simulink model "D_20210914_Modell_Inbetriebnahme_BreakOutBox_Jetson"  (R2021a)
settings: Solver=ode1  StartTime=0.0  StopTime=500  FixedStep=Ts  RelTol=1e-3
PreLoadFcn:
  | pulsePeriod = 0.05;
  | 
  | Ts = 0.001;
  | 
  | FPGA_Frequency = 75000000;
  | 
  | ts_IO691 = 5e-3;
PostLoadFcn:
  | ewolfSetUp
InitFcn:
  | pulsePeriod = 0.05;
  | 
  | Ts = 0.001;
  | 
  | FPGA_Frequency = 75000000;
  | 
  | ts_IO691 = 5e-3;
StopFcn:
  | Simulink.sdi.clearPreferences;
  | if isfile(['sdi_view_',bdroot,'.mldatx'])
  | Simulink.sdi.view;
  | pause(3);
  | Simulink.sdi.loadView(['sdi_view_',bdroot,]);
  | end
values from neighbouring files (symbols this model uses):
  max_ac = 2    [ewolfSetUp.m]
  max_steer = 0.26    [ewolfSetUp.m]
  min_ac = -3    [ewolfSetUp.m]
  min_steer = -0.26    [ewolfSetUp.m]
  PredictionHorizon = 30    [ewolfSetUp.m]
undefined symbols (not defined in the file or in its folder): canChannel, DiscIntNeverNeededParam, Ended, HS, IO291, IO397, Single
libraries: lllalib x255, canmsglib x143, simulink x33, speedgoatlib_IO191 x5, speedgoatlib_IO291 x5, speedgoatlib_IO691 x3, slrealtimeiplib x2, simulink_extras x1, speedgoatlib_fpga_dio x1, speedgoatlib_fpga_quadrature x1, speedgoatlib_fpga x1, canlib x1
(part 2 of 7)

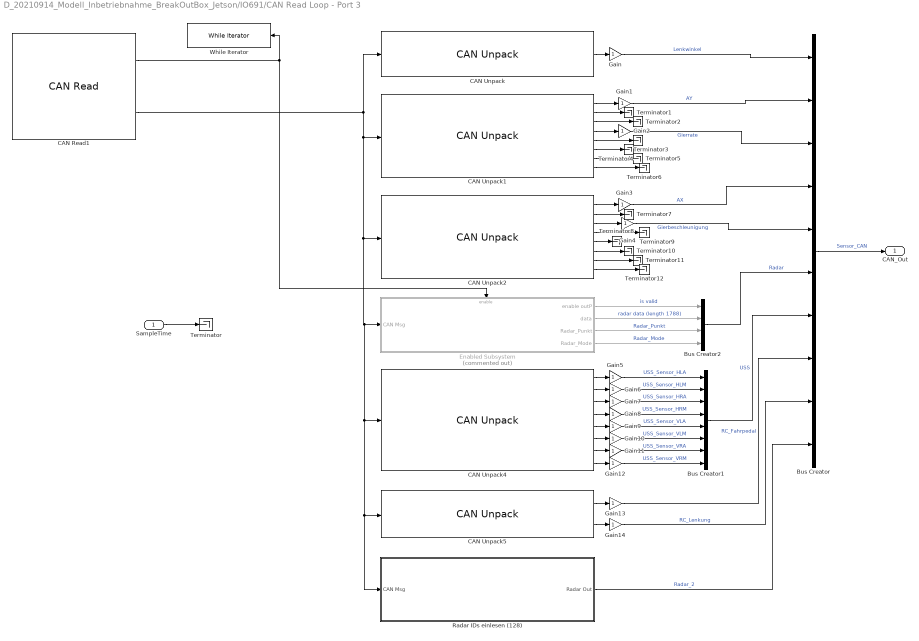
== system D_20210914_Modell_Inbetriebnahme_BreakOutBox_Jetson/IO691/CAN Read Loop - Port 3 ==
  SampleTime : Inport
  Bus Creator : BusCreator  Inputs=10
  Bus Creator1 : BusCreator  Inputs=8
  Bus Creator2 : BusCreator  Inputs=4
  CAN Read1 : speedgoatlib_IO691/CAN Read  id=1  ts=-1  channel=1  messageType=CAN  canType=CAN (HS)  BusOutput=off  initValues=[691 1 -1 0 1 1 0]
      settings: SourceProductName=Simulink Real-Time: Speedgoat Library
  CAN Unpack : canmsglib/CAN Unpack  CANdbFile=eWolf_SensorCAN.dbc  MsgList=Lenkwinkelsensor  MsgName=Lenkwinkelsensor  MsgIDType=Standard (11-bit identifier)  MsgIdentifier=2  MsgLength=2  SignalInfo={'Lenkwinkel','0','16','LE','signed','Standard','0','0.09882','0','-630','630'}  IDPort=off  TimestampPort=off  ErrorPort=off  RemotePort=off  LengthPort=off  StatusPort=off  ApplyMinMax=off
      settings: SourceProductBaseCode=ME,XP,VN  DataFormat=CANdb specified signals
  CAN Unpack1 : canmsglib/CAN Unpack  CANdbFile=eWolf_SensorCAN.dbc  MsgList=Beschleunigungssensor  MsgName=Beschleunigungssensor  MsgIDType=Standard (11-bit identifier)  MsgIdentifier=304  MsgLength=8  SignalInfo={'AY1','32','16','LE','unsigned','Standard','0','0.0001274','-4.1768','-4.1768','4.1768';'AY1_STAT','48','4','LE','unsigned','Standard','0','1','0','0','15';'CLU_STAT','16','4','LE','unsigned','Standard','0','1','0','0','15';'Gierrate','0','16','LE','unsigned','Standard','0','0.005','-163.84','-163.84','163.84';'Gierrate_STAT','52','4','LE','unsigned','Standard','0','1','0','0','15';'PSIP1_EXT_STAT','24','8','LE','unsigned','Standard','0','1','0','0','255';'TX1_CRC','56','8','LE','unsigned','Standard','0','1','0','0','255';'TX1_MSG_CNT','20','4','LE','unsigned','Standard','0','1','0','0','15'}  IDPort=off  TimestampPort=off  ErrorPort=off  RemotePort=off  LengthPort=off  StatusPort=off  ApplyMinMax=off
      settings: SourceProductBaseCode=ME,XP,VN  DataFormat=CANdb specified signals
  CAN Unpack2 : canmsglib/CAN Unpack  CANdbFile=eWolf_SensorCAN.dbc  MsgList=Beschleunigungssensor_2  MsgName=Beschleunigungssensor_2  MsgIDType=Standard (11-bit identifier)  MsgIdentifier=305  MsgLength=8  SignalInfo={'AX1','32','16','LE','unsigned','Standard','0','0.0001274','-4.1768','-4.1768','4.1768';'AX1_STAT','52','4','LE','unsigned','Standard','0','1','0','0','15';'Gierbeschleunigung','0','16','LE','unsigned','Standard','0','0.125','-4096','-4096','4096';'Gierbeschleunigung_STAT','20','4','LE','unsigned','Standard','0','1','0','0','15';'TX2_CRC','56','8','LE','unsigned','Standard','0','1','0','0','255';'TX2_MSG_CNT','48','4','LE','unsigned','Standard','0','1','0','0','15';'TX2_RES1','16','4','LE','unsigned','Standard','0','1','0','0','15';'TX2_RES2','24','8','LE','unsigned','Standard','0','1','0','0','255'}  IDPort=off  TimestampPort=off  ErrorPort=off  RemotePort=off  LengthPort=off  StatusPort=off  ApplyMinMax=off
      settings: SourceProductBaseCode=ME,XP,VN  DataFormat=CANdb specified signals
  CAN Unpack4 : canmsglib/CAN Unpack  CANdbFile=eWolf_SensorCAN.dbc  MsgList=Ultraschallsystem  MsgName=Ultraschallsystem  MsgIDType=Standard (11-bit identifier)  MsgIdentifier=16  MsgLength=8  SignalInfo={'USS_Sensor_HLA','32','8','LE','unsigned','Standard','0','1','0','0','255';'USS_Sensor_HLM','40','8','LE','unsigned','Standard','0','1','0','0','255';'USS_Sensor_HRA','56','8','LE','unsigned','Standard','0','1','0','0','255';'USS_Sensor_HRM','48','8','LE','unsigned','Standard','0','1','0','0','255';'USS_Sensor_VLA','0','8','LE','unsigned','Standard','0','1','0','0','255';'USS_Sensor_VLM','8','8','LE','unsigned','Standard','0','1','0','0','255';'USS_Sensor_VRA','24','8','LE','unsigned','Standard','0','1','0','0','255';'USS_Sensor_VRM','16','8','LE','unsigned','Standard','0','1','0','0','255'}  IDPort=off  TimestampPort=off  ErrorPort=off  RemotePort=off  LengthPort=off  StatusPort=off  ApplyMinMax=off
      settings: SourceProductBaseCode=ME,XP,VN  DataFormat=CANdb specified signals
  CAN Unpack5 : canmsglib/CAN Unpack  CANdbFile=eWolf_SensorCAN.dbc  MsgList=RC_Fernsteuerung  MsgName=RC_Fernsteuerung  MsgIDType=Standard (11-bit identifier)  MsgIdentifier=17  MsgLength=2  SignalInfo={'RC_Fahrpedal','8','8','LE','unsigned','Standard','0','1','0','0','255';'RC_Lenkung','0','8','LE','unsigned','Standard','0','1','0','0','255'}  IDPort=off  TimestampPort=off  ErrorPort=off  RemotePort=off  LengthPort=off  StatusPort=off  ApplyMinMax=off
      settings: SourceProductBaseCode=ME,XP,VN  DataFormat=CANdb specified signals
  Enabled Subsystem : Subsystem  Commented=on  TreatAsAtomicUnit=on
  Gain{,1..14} (15 alike) : Gain
  Radar IDs einlesen (128) : Subsystem
  Terminator{,1..12} (13 alike) : Terminator
  While Iterator : WhileIterator  MaxIters=501  WhileBlockType=do-while
  CAN_Out : Outport
  wires:
  SampleTime/1 -> Terminator/1
  CAN Read1/1 -> Enabled Subsystem/Enable, While Iterator/1
  CAN Read1/2 -> CAN Unpack/1, Radar IDs einlesen (128)/1(CAN Msg), CAN Unpack5/1, CAN Unpack4/1, Enabled Subsystem/1(CAN Msg), CAN Unpack2/1, CAN Unpack1/1
  Bus Creator/1 -> CAN_Out/1  "Sensor_CAN"
  CAN Unpack/1 -> Gain/1
  CAN Unpack1/1 -> Gain1/1
  CAN Unpack1/5 -> Terminator3/1
  CAN Unpack2/1 -> Gain3/1
  CAN Unpack2/5 -> Terminator8/1
  CAN Unpack1/2 -> Terminator1/1
  CAN Unpack1/3 -> Terminator2/1
  CAN Unpack1/4 -> Gain2/1
  CAN Unpack1/6 -> Terminator4/1
  CAN Unpack1/7 -> Terminator5/1
  CAN Unpack1/8 -> Terminator6/1
  Gain/1 -> Bus Creator/1  "Lenkwinkel"
  Gain1/1 -> Bus Creator/2  "AY"
  Gain2/1 -> Bus Creator/3  "Gierrate"
  Gain3/1 -> Bus Creator/4  "AX"
  Gain4/1 -> Bus Creator/5  "Gierbeschleunigung"
  CAN Unpack2/2 -> Terminator7/1
  CAN Unpack2/3 -> Gain4/1
  CAN Unpack2/4 -> Terminator9/1
  CAN Unpack2/6 -> Terminator10/1
  CAN Unpack2/7 -> Terminator11/1
  CAN Unpack2/8 -> Terminator12/1
  CAN Unpack4/1 -> Gain5/1
  CAN Unpack4/2 -> Gain6/1
  CAN Unpack4/3 -> Gain7/1
  CAN Unpack4/4 -> Gain8/1
  CAN Unpack4/5 -> Gain9/1
  CAN Unpack4/6 -> Gain10/1
  CAN Unpack4/7 -> Gain11/1
  CAN Unpack4/8 -> Gain12/1
  Gain5/1 -> Bus Creator1/1  "USS_Sensor_HLA"
  Gain6/1 -> Bus Creator1/2  "USS_Sensor_HLM"
  Gain7/1 -> Bus Creator1/3  "USS_Sensor_HRA"
  Gain8/1 -> Bus Creator1/4  "USS_Sensor_HRM"
  Gain9/1 -> Bus Creator1/5  "USS_Sensor_VLA"
  Gain10/1 -> Bus Creator1/6  "USS_Sensor_VLM"
  Gain11/1 -> Bus Creator1/7  "USS_Sensor_VRA"
  Gain12/1 -> Bus Creator1/8  "USS_Sensor_VRM"
  Bus Creator1/1 -> Bus Creator/7  "USS"
  CAN Unpack5/1 -> Gain13/1
  CAN Unpack5/2 -> Gain14/1
  Gain13/1 -> Bus Creator/8  "RC_Fahrpedal"
  Gain14/1 -> Bus Creator/9  "RC_Lenkung"
  Enabled Subsystem/1(enable outP) -> Bus Creator2/1  "is valid"
  Enabled Subsystem/2(data) -> Bus Creator2/2  "radar data (length 1788)"
  Enabled Subsystem/3(Radar_Punkt) -> Bus Creator2/3  "Radar_Punkt"
  Enabled Subsystem/4(Radar_Mode) -> Bus Creator2/4  "Radar_Mode"
  Bus Creator2/1 -> Bus Creator/6  "Radar"
  Radar IDs einlesen (128)/1(Radar Out) -> Bus Creator/10  "Radar_2"

== system D_20210914_Modell_Inbetriebnahme_BreakOutBox_Jetson/Nvidia_Jetson/LaneFollowingAndControl ==
  Set velocity : Inport
  Longitudinal_Velocity : Inport  Port=2
  Lane Detections : Inport  Port=3
  Estimate Lane Center1 : Subsystem  VariantControl=v2
  MPC Controller : Subsystem
  steering_angle : Outport
  acceleration : Outport  Port=2
  wires:
  Longitudinal_Velocity/1 -> MPC Controller/2(Longitudinal velocity), Estimate Lane Center1/2(Longitudinal Velocity)
  MPC Controller/2(Acceleration) -> acceleration/1  "acceleration"
  Estimate Lane Center1/2(Lateral Offset) -> MPC Controller/4(Lateral deviation)  "lateral_deviation"
  Estimate Lane Center1/1(Previewed Curvature) -> MPC Controller/3(Curvature)  "previewed_curvature"
  Estimate Lane Center1/3(Heading Angle) -> MPC Controller/5(Relative yaw angle)  "relative_yaw_angle"
  Set velocity/1 -> MPC Controller/1(Set velocity)
  MPC Controller/1(Steering Angle) -> steering_angle/1  "steering_angle"
  Lane Detections/1 -> Estimate Lane Center1/1(Lane Detections)

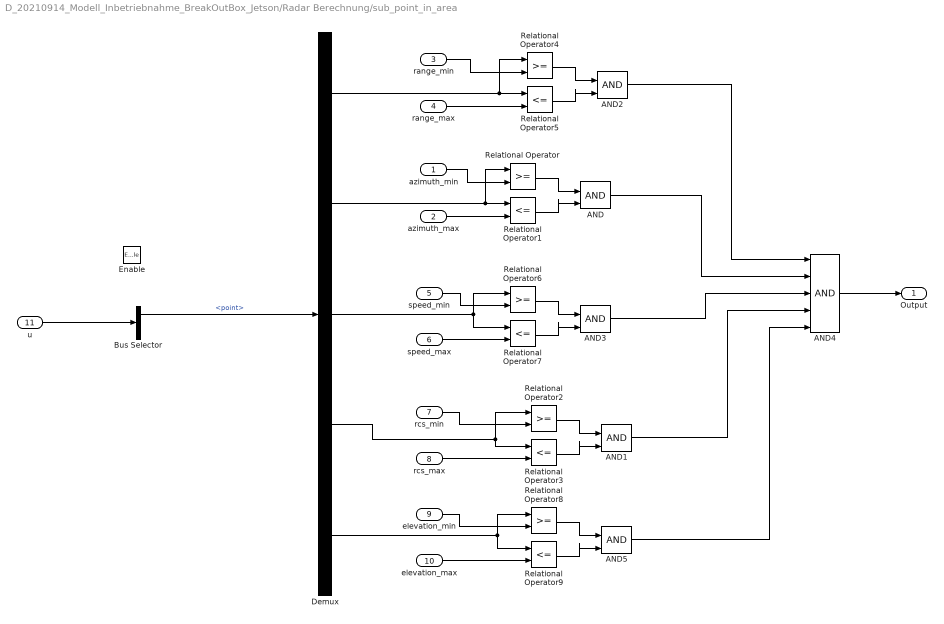
== system D_20210914_Modell_Inbetriebnahme_BreakOutBox_Jetson/Radar Berechnung/sub_point_in_area ==
  azimuth_min : Inport
  azimuth_max : Inport  Port=2
  range_min : Inport  Port=3
  range_max : Inport  Port=4
  speed_min : Inport  Port=5
  speed_max : Inport  Port=6
  rcs_min : Inport  Port=7
  rcs_max : Inport  Port=8
  elevation_min : Inport  Port=9
  elevation_max : Inport  Port=10
  u : Inport  Port=11
  Enable : EnablePort
  AND{,1..3,5} (5 alike) : Logic  IconShape=distinctive  AllPortsSameDT=off  OutDataTypeStr=boolean
  AND4 : Logic  Inputs=5  IconShape=distinctive  AllPortsSameDT=off  OutDataTypeStr=boolean
  Bus Selector : BusSelector  OutputSignals=point,CANID
  Demux : Demux  Outputs=5
  Relational Operator{,2,4,6,8} (5 alike) : RelationalOperator  OutDataTypeStr=boolean  RndMeth=Simplest
  Relational Operator{1,3,5,7,9} (5 alike) : RelationalOperator  Operator=<=  OutDataTypeStr=boolean  RndMeth=Simplest
  Output : Outport
  wires:
  Demux/5 -> Relational Operator8/1, Relational Operator9/1
  Demux/4 -> Relational Operator3/1, Relational Operator2/1
  Demux/3 -> Relational Operator6/1, Relational Operator7/1
  Demux/1 -> Relational Operator5/1, Relational Operator4/1
  Demux/2 -> Relational Operator1/1, Relational Operator/1
  elevation_max/1 -> Relational Operator9/2
  AND5/1 -> AND4/5
  Relational Operator8/1 -> AND5/1
  Relational Operator9/1 -> AND5/2
  elevation_min/1 -> Relational Operator8/2
  range_min/1 -> Relational Operator4/2
  azimuth_min/1 -> Relational Operator/2
  speed_min/1 -> Relational Operator6/2
  rcs_min/1 -> Relational Operator2/2
  Relational Operator6/1 -> AND3/1
  Relational Operator/1 -> AND/1
  AND4/1 -> Output/1
  Relational Operator4/1 -> AND2/1
  Relational Operator2/1 -> AND1/1
  Relational Operator5/1 -> AND2/2
  Relational Operator3/1 -> AND1/2
  Relational Operator7/1 -> AND3/2
  speed_max/1 -> Relational Operator7/2
  Relational Operator1/1 -> AND/2
  AND2/1 -> AND4/1
  u/1 -> Bus Selector/1
  AND/1 -> AND4/2
  AND1/1 -> AND4/4
  Bus Selector/1 -> Demux/1  "<point>"
  rcs_max/1 -> Relational Operator3/2
  range_max/1 -> Relational Operator5/2
  AND3/1 -> AND4/3
  azimuth_max/1 -> Relational Operator1/2

== system D_20210914_Modell_Inbetriebnahme_BreakOutBox_Jetson/Bremspedal Steuerung/QAD Steuerung1/Anti-Relaisprellen ==
  In : Inport
  Bias : Bias  Bias=-Ts
  Compare To Zero : simulink/Logic and Bit Operations/Compare To Zero  relop===  OutDataTypeStr=boolean
  Constant : Constant  Value=0.2
  Constant1 : Constant  Value=0
  Delay1 : Delay  DelayLength=1  InputProcessing=Columns as channels (frame based)
  Detect Increase : simulink/Logic and Bit Operations/Detect Increase  vinit=0.0  OutDataTypeStr=boolean
  Saturation : Saturate  UpperLimit=0.2  LowerLimit=0
  Switch : Switch  Criteria=u2 ~= 0
  Switch1 : Switch  Criteria=u2 ~= 0
  Out : Outport  VectorParamsAs1DForOutWhenUnconnected=off
  wires:
  Compare To Zero/1 -> Switch1/2
  In/1 -> Detect Increase/1, Switch1/1
  Switch1/1 -> Out/1
  Constant1/1 -> Switch1/3
  Delay1/1 -> Bias/1, Compare To Zero/1
  Constant/1 -> Switch/1
  Detect Increase/1 -> Switch/2
  Switch/1 -> Delay1/1
  Bias/1 -> Saturation/1
  Saturation/1 -> Switch/3

== system D_20210914_Modell_Inbetriebnahme_BreakOutBox_Jetson/Bremspedal Steuerung/QAD Steuerung1/Counter ==
  count_dir : Inport
  count_enable : Inport  Port=2
  AND5 : Logic  AllPortsSameDT=off  OutDataTypeStr=boolean
  AND6 : Logic  AllPortsSameDT=off  OutDataTypeStr=boolean
  Add : Sum
  Compare To Constant5 : simulink/Logic and Bit Operations/Compare To Constant  relop===  const=1  OutDataTypeStr=boolean
  Compare To Zero : simulink/Logic and Bit Operations/Compare To Zero  relop=>  OutDataTypeStr=boolean
  Compare To Zero1 : simulink/Logic and Bit Operations/Compare To Zero  relop===  OutDataTypeStr=boolean
  Constant : Constant  Value=-1
  Constant1 : Constant  Value=0
  Constant2 : Constant
  Switch : Switch  Criteria=u2 > Threshold
  Switch1 : Switch  Criteria=u2 > Threshold
  Unit Delay : UnitDelay  SampleTime=-1  HasFrameUpgradeWarning=on
  Value : Outport
  wires:
  count_dir/1 -> Compare To Zero1/1, Compare To Constant5/1
  Compare To Zero/1 -> AND6/2, AND5/2
  Constant1/1 -> Switch/3
  AND6/1 -> Switch1/2
  Switch1/1 -> Add/1
  AND5/1 -> Switch/2
  Switch/1 -> Switch1/3
  Compare To Constant5/1 -> AND5/1
  Constant2/1 -> Switch1/1
  Compare To Zero1/1 -> AND6/1
  Constant/1 -> Switch/1
  Unit Delay/1 -> Add/2
  count_enable/1 -> Compare To Zero/1
  Add/1 -> Value/1, Unit Delay/1

== system D_20210914_Modell_Inbetriebnahme_BreakOutBox_Jetson/Bremspedal Steuerung/QAD Steuerung1/QAD1 ==
  Hall_A : Inport
  Hall_B : Inport  Port=2
  Data Type Conversion : DataTypeConversion
  Data Type Conversion1 : DataTypeConversion
  State Transition Table : State Transition Table  TreatAsAtomicUnit=on
  Count_direction : Outport
  Count_enable : Outport  Port=2
  wires:
  Hall_A/1 -> Data Type Conversion/1
  Hall_B/1 -> Data Type Conversion1/1
  Data Type Conversion/1 -> State Transition Table/1(Hall_A)
  Data Type Conversion1/1 -> State Transition Table/2(Hall_B)
  State Transition Table/1(count_enable) -> Count_enable/1
  State Transition Table/2(count_dir) -> Count_direction/1

== system D_20210914_Modell_Inbetriebnahme_BreakOutBox_Jetson/Freigabe/Freigabe/1s Tastersperre ==
  In : Inport
  Bias : Bias  Bias=-Ts
  Compare To Zero : simulink/Logic and Bit Operations/Compare To Zero  relop===  OutDataTypeStr=boolean
  Constant : Constant
  Constant1 : Constant  Value=0
  Delay1 : Delay  DelayLength=1  InputProcessing=Columns as channels (frame based)
  Detect Increase : simulink/Logic and Bit Operations/Detect Increase  vinit=0.0  OutDataTypeStr=boolean
  Saturation : Saturate  UpperLimit=1  LowerLimit=0
  Switch : Switch  Criteria=u2 ~= 0
  Switch1 : Switch  Criteria=u2 ~= 0
  Out : Outport  VectorParamsAs1DForOutWhenUnconnected=off
  wires:
  Compare To Zero/1 -> Switch1/2
  In/1 -> Detect Increase/1, Switch1/1
  Switch1/1 -> Out/1
  Constant1/1 -> Switch1/3
  Delay1/1 -> Bias/1, Compare To Zero/1
  Constant/1 -> Switch/1
  Detect Increase/1 -> Switch/2
  Switch/1 -> Delay1/1
  Bias/1 -> Saturation/1
  Saturation/1 -> Switch/3

== system D_20210914_Modell_Inbetriebnahme_BreakOutBox_Jetson/Freigabe/Freigabe/Detektion Fahrpedal ==
  FP_1_In : Inport
  FP_2_In : Inport  Port=2
  AND : Logic  AllPortsSameDT=off  OutDataTypeStr=boolean
  Compare To Constant : simulink/Logic and Bit Operations/Compare To Constant  relop=<=  const=1.1  OutDataTypeStr=boolean
  Compare To Constant1 : simulink/Logic and Bit Operations/Compare To Constant  relop=<=  const=0.7  OutDataTypeStr=boolean
  Moving Average : Subsystem
  Moving Average1 : Subsystem
  FP_Freigabe : Outport
  wires:
  FP_1_In/1 -> Moving Average/1(In)
  FP_2_In/1 -> Moving Average1/1(In)
  AND/1 -> FP_Freigabe/1
  Moving Average/1(Out) -> Compare To Constant/1
  Moving Average1/1(Out) -> Compare To Constant1/1
  Compare To Constant/1 -> AND/1
  Compare To Constant1/1 -> AND/2

== system D_20210914_Modell_Inbetriebnahme_BreakOutBox_Jetson/Freigabe/Freigabe/Detektion Lenkung ==
  note: Detektion Schwellwertüberschreitung (0,8)
  note: Dauer der Schwellwertüberschreitung > 0,2s?
  LG_1_In : Inport
  LG_2_In : Inport  Port=2
  Abs2 : Abs
  Compare To Constant4 : simulink/Logic and Bit Operations/Compare To Constant  relop=>  const=0.8  OutDataTypeStr=boolean
  Data Type Conversion2 : DataTypeConversion  OutDataTypeStr=double
  Delta_Time1 : Constant  Value=0.2
  Discrete-Time Integrator2 : DiscreteIntegrator  ExternalReset=falling  SampleTime=-1  ICPrevOutput=DiscIntNeverNeededParam  ICPrevScaledInput=DiscIntNeverNeededParam
  Relational Operator2 : RelationalOperator  Operator=<  OutDataTypeStr=boolean  RndMeth=Simplest
  Subtract2 : Sum  Inputs=+-
  LG_Freigabe : Outport
  wires:
  LG_1_In/1 -> Subtract2/1
  LG_2_In/1 -> Subtract2/2
  Relational Operator2/1 -> LG_Freigabe/1
  Subtract2/1 -> Abs2/1
  Abs2/1 -> Compare To Constant4/1
  Data Type Conversion2/1 -> Discrete-Time Integrator2/2, Discrete-Time Integrator2/1
  Compare To Constant4/1 -> Data Type Conversion2/1
  Discrete-Time Integrator2/1 -> Relational Operator2/1
  Delta_Time1/1 -> Relational Operator2/2

== system D_20210914_Modell_Inbetriebnahme_BreakOutBox_Jetson/Freigabe/Freigabe/EMV Filter ==
  In : Inport
  Compare To Constant : simulink/Logic and Bit Operations/Compare To Constant  relop===  const=1  OutDataTypeStr=boolean
  Divide : Product  Inputs=*/
  Sum of Elements : Sum  Inputs=+
  Tapped Delay1 : simulink/Discrete/Tapped Delay  vinit=0.0  samptime=-1  NumDelays=4  DelayOrder=Oldest  includeCurrent=off
  Vector Concatenate : Concatenate
  Width : Width
  Out : Outport  VectorParamsAs1DForOutWhenUnconnected=off
  wires:
  In/1 -> Vector Concatenate/1, Tapped Delay1/1
  Tapped Delay1/1 -> Vector Concatenate/2
  Vector Concatenate/1 -> Sum of Elements/1, Width/1
  Divide/1 -> Compare To Constant/1
  Sum of Elements/1 -> Divide/1
  Width/1 -> Divide/2
  Compare To Constant/1 -> Out/1

== system D_20210914_Modell_Inbetriebnahme_BreakOutBox_Jetson/IO691/CAN Read Loop - Port 3/Enabled Subsystem ==
  CAN Msg : Inport
  Enable : EnablePort
  extract radar data from CAN msg stream : Subsystem  Description=|
      | Extract radar data from CAN messages and create vector object with: 1788 fields:
      | 
      | 1. Timestamp
      | 2. cycle_count
      | 3. number of Objects
      | 4. radar timestamp_header
      | 5. CAN ID
      | +++++++++++++++++++++
      | % last point
      | 6. range
      | 7. az
      | 8. vr
      | 9. rcs
      | 10. el
      | ----------------------------------
      | % last point -1
      | 11. range
      | 12. az
      | 13. vr
      | 14. rcs
      | 15. el
      |  ...
      | 
      | empty points, all values == 0
  enable outP : Outport
  data : Outport  Port=2
  Radar_Punkt : Outport  Port=3
  Radar_Mode : Outport  Port=4
  wires:
  CAN Msg/1 -> extract radar data from CAN msg stream/1(msg)
  extract radar data from CAN msg stream/1(enable outP) -> enable outP/1
  extract radar data from CAN msg stream/2(data) -> data/1
  extract radar data from CAN msg stream/3(Radar_Punkt) -> Radar_Punkt/1
  extract radar data from CAN msg stream/4(Radar_Mode) -> Radar_Mode/1
